simulink model "hw4_p1"  (R2020a)
settings: Solver=VariableStepAuto  StartTime=0.0  StopTime=60  RelTol=1e-7
undefined symbols (not defined in the file or in its folder): A, A_pg, A_sp, B, B_pg, B_sp, C, C_pg, C_sp, D, D_pg, D_sp, IC, IC_pg, IC_sp
settings Model: Creator=Tomo  LastModifiedBy=Tomo

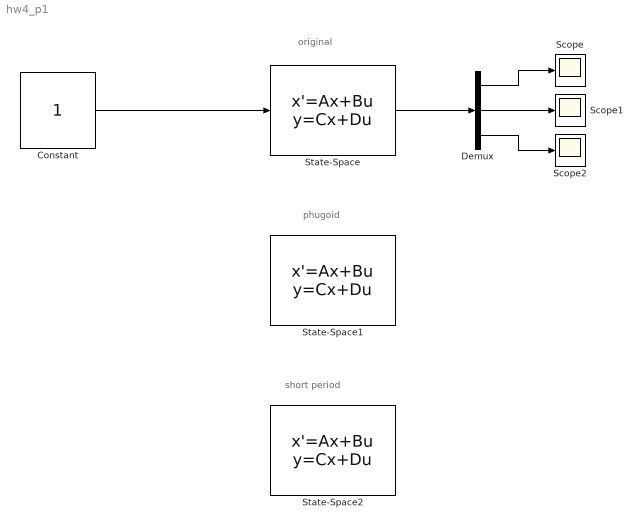
== system hw4_p1 ==
  note: original
  note: phugoid
  note: short period
  Constant : Constant
  Demux : Demux  Outputs=3
  Scope : Scope
  Scope1 : Scope
  Scope2 : Scope
  State-Space : StateSpace  A=A  B=B  C=C  D=D  InitialCondition=IC
  State-Space1 : StateSpace  A=A_pg  B=B_pg  C=C_pg  D=D_pg  InitialCondition=IC_pg
  State-Space2 : StateSpace  A=A_sp  B=B_sp  C=C_sp  D=D_sp  InitialCondition=IC_sp
  wires:
  Constant/1 -> State-Space/1
  State-Space/1 -> Demux/1
  Demux/1 -> Scope/1
  Demux/2 -> Scope1/1
  Demux/3 -> Scope2/1
